simulink model "MK_control_SIL_20200323"  (R2016b)
settings: Solver=ode4  StartTime=0.0  StopTime=inf  FixedStep=0.004  RelTol=1e-7
libraries: simulink x6, simulink_extras x3, etargetslib x1, dspnetwork x1, X_Plane_Communication_Library x1
settings Model: Creator=E6320  LastModifiedBy=user
settings SolverCC: AlgebraicLoopSolver=LineSearch
settings DataIOCC: SaveOutput=off  SignalLogging=off  DSMLogging=off  SaveTime=off

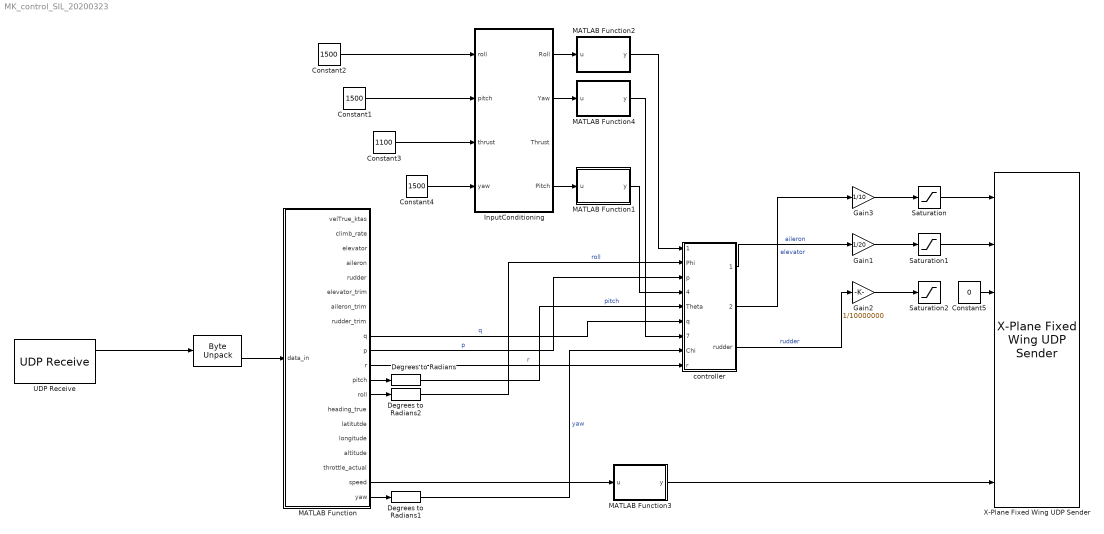
== system MK_control_SIL_20200323 ==
  "     " : etargetslib/Byte Unpack  dimensions={5,[9,21]}  datatypes={'uint8','single'}  byteAlign=1
  Constant1 : Constant  Value=1500
  Constant2 : Constant  Value=1500
  Constant3 : Constant  Value=1100
  Constant4 : Constant  Value=1500
  Constant5 : Constant  Value=0
  Degrees to Radians : simulink_extras/Transformations/Degrees to Radians
  Degrees to Radians1 : simulink_extras/Transformations/Degrees to Radians
  Degrees to Radians2 : simulink_extras/Transformations/Degrees to Radians
  Gain1 : Gain  Gain=1/20
  Gain2 : Gain  Gain=1/10000000
  Gain3 : Gain  Gain=1/10
  InputConditioning : Subsystem
  MATLAB Function : MATLAB Function  TreatAsAtomicUnit=on
  MATLAB Function1 : MATLAB Function  TreatAsAtomicUnit=on
  MATLAB Function2 : MATLAB Function  TreatAsAtomicUnit=on
  MATLAB Function3 : MATLAB Function  TreatAsAtomicUnit=on
  MATLAB Function4 : MATLAB Function  TreatAsAtomicUnit=on
  Saturation : Saturate  UpperLimit=1  LowerLimit=-1
  Saturation1 : Saturate  UpperLimit=1  LowerLimit=-1
  Saturation2 : Saturate  UpperLimit=1  LowerLimit=-1
  UDP Receive : dspnetwork/UDP Receive  localURL='0.0.0.0'  localPort=49005  remoteURL='127.0.0.1'  remotePort=-1  recvBufferSize=8192  dims=761  signalDatatype=uint8  isVarSize=off  showBlockingTime=on  blockingTime=10  sampletime=0.02  blockPlatform=HOST
  X-Plane Fixed Wing UDP Sender : X_Plane_Communication_Library/Fixed Wing/X-Plane Fixed Wing UDP Sender  ip_adress='127.0.0.1'  port_number=49000
  "controller " : Subsystem
  wires:
  UDP Receive/1 -> "     "/1
  "     "/2 -> MATLAB Function/1(data_in)
  Constant3/1 -> InputConditioning/3(thrust)
  Constant4/1 -> InputConditioning/4(yaw)
  Constant2/1 -> InputConditioning/1(roll)
  Constant1/1 -> InputConditioning/2(pitch)
  InputConditioning/4("Pitch ") -> MATLAB Function1/1(u)
  InputConditioning/1(Roll) -> MATLAB Function2/1(u)
  InputConditioning/2(Yaw) -> MATLAB Function4/1(u)
  MATLAB Function/19(speed) -> MATLAB Function3/1(u)
  MATLAB Function3/1(y) -> X-Plane Fixed Wing UDP Sender/7
  MATLAB Function/12(pitch) -> Degrees to Radians/1
  MATLAB Function/13(roll) -> Degrees to Radians2/1
  Saturation/1 -> X-Plane Fixed Wing UDP Sender/1
  Saturation1/1 -> X-Plane Fixed Wing UDP Sender/2
  MATLAB Function2/1(y) -> "controller "/1(PhiCmd)
  MATLAB Function4/1(y) -> "controller "/7(ChiCmd)
  MATLAB Function1/1(y) -> "controller "/4(ThetaCmd)
  MATLAB Function/9(q) -> "controller "/6(q)  "q"
  MATLAB Function/10(p) -> "controller "/3(p)  "p"
  MATLAB Function/11(r) -> "controller "/9(r)  "r"
  Degrees to Radians/1 -> "controller "/5(Theta)  "pitch"
  Degrees to Radians2/1 -> "controller "/2(Phi)  "roll"
  Degrees to Radians1/1 -> "controller "/8(Chi)  "yaw"
  "controller "/1(aileron) -> Gain1/1  "aileron"
  "controller "/3(rudder) -> Gain2/1  "rudder"
  "controller "/2(elevator) -> Gain3/1  "elevator"
  Gain3/1 -> Saturation/1
  Gain1/1 -> Saturation1/1
  Gain2/1 -> Saturation2/1
  MATLAB Function/20(yaw) -> Degrees to Radians1/1
  Constant5/1 -> X-Plane Fixed Wing UDP Sender/3

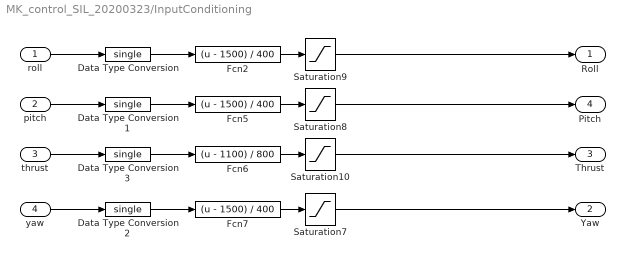
== system MK_control_SIL_20200323/InputConditioning ==
  roll : Inport
  pitch : Inport  Port=2
  thrust : Inport  Port=3
  yaw : Inport  Port=4
  Data Type Conversion{,1..3} (4 alike) : DataTypeConversion  OutDataTypeStr=single
  Fcn2 : Fcn  Expr=(u - 1500) / 400
  Fcn5 : Fcn  Expr=(u - 1500) / 400
  Fcn6 : Fcn  Expr=(u - 1100) / 800
  Fcn7 : Fcn  Expr=(u - 1500) / 400
  Saturation10 : Saturate  UpperLimit=1  LowerLimit=0
  Saturation7 : Saturate  UpperLimit=1  LowerLimit=-1
  Saturation8 : Saturate  UpperLimit=1  LowerLimit=-1
  Saturation9 : Saturate  UpperLimit=1  LowerLimit=-1
  Roll : Outport
  Yaw : Outport  Port=2
  Thrust : Outport  Port=3
  "Pitch " : Outport  Port=4
  wires:
  Saturation10/1 -> Thrust/1
  Saturation9/1 -> Roll/1
  Fcn6/1 -> Saturation10/1
  thrust/1 -> Data Type Conversion3/1
  Fcn2/1 -> Saturation9/1
  Fcn5/1 -> Saturation8/1
  Fcn7/1 -> Saturation7/1
  yaw/1 -> Data Type Conversion2/1
  pitch/1 -> Data Type Conversion1/1
  roll/1 -> Data Type Conversion/1
  Data Type Conversion/1 -> Fcn2/1
  Data Type Conversion1/1 -> Fcn5/1
  Data Type Conversion2/1 -> Fcn7/1
  Data Type Conversion3/1 -> Fcn6/1
  Saturation8/1 -> "Pitch "/1
  Saturation7/1 -> Yaw/1

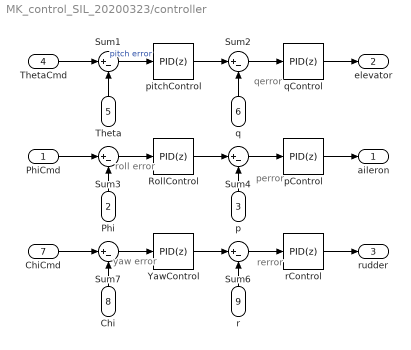
== system MK_control_SIL_20200323/controller  ==
  note: rerror
  note: yaw error
  note: roll error
  note: perror
  note: qerror
  PhiCmd : Inport
  Phi : Inport  Port=2
  p : Inport  Port=3
  ThetaCmd : Inport  Port=4
  Theta : Inport  Port=5
  q : Inport  Port=6
  ChiCmd : Inport  Port=7
  Chi : Inport  Port=8
  r : Inport  Port=9
  RollControl : simulink/Continuous/PID Controller  Controller=PID  TimeDomain=Discrete-time  SampleTime=0.004  IntegratorMethod=Forward Euler  FilterMethod=Forward Euler  Form=Parallel  UseFilter=on  ControllerParametersSource=internal  P=4.82  I=0.5842424242  D=0.401024  N=20.6  InitialConditionSource=internal  InitialConditionForIntegrator=0  InitialConditionForFilter=0  ExternalReset=none  LimitOutput=off  UpperSaturationLimit=inf  LowerSaturationLimit=-inf  LinearizeAsGain=on  AntiWindupMode=none  Kb=1  TrackingMode=off  Kt=1  PParamMin=[]  PParamMax=[]  IParamMin=[]  IParamMax=[]  DParamMin=[]  DParamMax=[]  NParamMin=[]  NParamMax=[]  KbParamMin=[]  KbParamMax=[]  KtParamMin=[]  KtParamMax=[]  POutMin=[]  POutMax=[]  IOutMin=[]  IOutMax=[]  DOutMin=[]  DOutMax=[]  NOutMin=[]  NOutMax=[]  KbOutMin=[]  KbOutMax=[]  KtOutMin=[]  KtOutMax=[]  IntegratorOutMin=[]  IntegratorOutMax=[]  FilterOutMin=[]  FilterOutMax=[]  SumOutMin=[]  SumOutMax=[]  SumI1OutMin=[]  SumI1OutMax=[]  SumI2OutMin=[]  SumI2OutMax=[]  SumI3OutMin=[]  SumI3OutMax=[]  SumDOutMin=[]  SumDOutMax=[]  SaturationOutMin=[]  SaturationOutMax=[]  IntegratorContinuousStateAttributes=''  IntegratorStateMustResolveToSignalObject=off  IntegratorRTWStateStorageClass=Auto  FilterContinuousStateAttributes=''  FilterStateMustResolveToSignalObject=off  FilterRTWStateStorageClass=Auto  DifferentiatorICPrevScaledInput=0  DifferentiatorOutMin=[]  DifferentiatorOutMax=[]
  Sum{1..4,6..7} (6 alike) : Sum  Inputs=|+-
  YawControl : simulink/Continuous/PID Controller  Controller=PID  TimeDomain=Discrete-time  SampleTime=0.004  IntegratorMethod=Forward Euler  FilterMethod=Forward Euler  Form=Parallel  UseFilter=on  ControllerParametersSource=internal  P=17.9  I=36.30831643  D=0.24881  N=3.48  InitialConditionSource=internal  InitialConditionForIntegrator=0  InitialConditionForFilter=0  ExternalReset=none  LimitOutput=off  UpperSaturationLimit=inf  LowerSaturationLimit=-inf  LinearizeAsGain=on  AntiWindupMode=none  Kb=1  TrackingMode=off  Kt=1  PParamMin=[]  PParamMax=[]  IParamMin=[]  IParamMax=[]  DParamMin=[]  DParamMax=[]  NParamMin=[]  NParamMax=[]  KbParamMin=[]  KbParamMax=[]  KtParamMin=[]  KtParamMax=[]  POutMin=[]  POutMax=[]  IOutMin=[]  IOutMax=[]  DOutMin=[]  DOutMax=[]  NOutMin=[]  NOutMax=[]  KbOutMin=[]  KbOutMax=[]  KtOutMin=[]  KtOutMax=[]  IntegratorOutMin=[]  IntegratorOutMax=[]  FilterOutMin=[]  FilterOutMax=[]  SumOutMin=[]  SumOutMax=[]  SumI1OutMin=[]  SumI1OutMax=[]  SumI2OutMin=[]  SumI2OutMax=[]  SumI3OutMin=[]  SumI3OutMax=[]  SumDOutMin=[]  SumDOutMax=[]  SaturationOutMin=[]  SaturationOutMax=[]  IntegratorContinuousStateAttributes=''  IntegratorStateMustResolveToSignalObject=off  IntegratorRTWStateStorageClass=Auto  FilterContinuousStateAttributes=''  FilterStateMustResolveToSignalObject=off  FilterRTWStateStorageClass=Auto  DifferentiatorICPrevScaledInput=0  DifferentiatorOutMin=[]  DifferentiatorOutMax=[]
  pControl : simulink/Continuous/PID Controller  Controller=PID  TimeDomain=Discrete-time  SampleTime=0.004  IntegratorMethod=Forward Euler  FilterMethod=Forward Euler  Form=Parallel  UseFilter=on  ControllerParametersSource=internal  P=0.302  I=2.770642202  D=0.0097546  N=8.07  InitialConditionSource=internal  InitialConditionForIntegrator=0  InitialConditionForFilter=0  ExternalReset=none  LimitOutput=off  UpperSaturationLimit=inf  LowerSaturationLimit=-inf  LinearizeAsGain=on  AntiWindupMode=none  Kb=1  TrackingMode=off  Kt=1  PParamMin=[]  PParamMax=[]  IParamMin=[]  IParamMax=[]  DParamMin=[]  DParamMax=[]  NParamMin=[]  NParamMax=[]  KbParamMin=[]  KbParamMax=[]  KtParamMin=[]  KtParamMax=[]  POutMin=[]  POutMax=[]  IOutMin=[]  IOutMax=[]  DOutMin=[]  DOutMax=[]  NOutMin=[]  NOutMax=[]  KbOutMin=[]  KbOutMax=[]  KtOutMin=[]  KtOutMax=[]  IntegratorOutMin=[]  IntegratorOutMax=[]  FilterOutMin=[]  FilterOutMax=[]  SumOutMin=[]  SumOutMax=[]  SumI1OutMin=[]  SumI1OutMax=[]  SumI2OutMin=[]  SumI2OutMax=[]  SumI3OutMin=[]  SumI3OutMax=[]  SumDOutMin=[]  SumDOutMax=[]  SaturationOutMin=[]  SaturationOutMax=[]  IntegratorContinuousStateAttributes=''  IntegratorStateMustResolveToSignalObject=off  IntegratorRTWStateStorageClass=Auto  FilterContinuousStateAttributes=''  FilterStateMustResolveToSignalObject=off  FilterRTWStateStorageClass=Auto  DifferentiatorICPrevScaledInput=0  DifferentiatorOutMin=[]  DifferentiatorOutMax=[]
  pitchControl : simulink/Continuous/PID Controller  Controller=PID  TimeDomain=Discrete-time  SampleTime=0.004  IntegratorMethod=Forward Euler  FilterMethod=Forward Euler  Form=Parallel  UseFilter=on  ControllerParametersSource=internal  P=5.91  I=5.91  D=0.19503  N=8.24  InitialConditionSource=internal  InitialConditionForIntegrator=0  InitialConditionForFilter=0  ExternalReset=none  LimitOutput=off  UpperSaturationLimit=inf  LowerSaturationLimit=-inf  LinearizeAsGain=on  AntiWindupMode=none  Kb=1  TrackingMode=off  Kt=1  PParamMin=[]  PParamMax=[]  IParamMin=[]  IParamMax=[]  DParamMin=[]  DParamMax=[]  NParamMin=[]  NParamMax=[]  KbParamMin=[]  KbParamMax=[]  KtParamMin=[]  KtParamMax=[]  POutMin=[]  POutMax=[]  IOutMin=[]  IOutMax=[]  DOutMin=[]  DOutMax=[]  NOutMin=[]  NOutMax=[]  KbOutMin=[]  KbOutMax=[]  KtOutMin=[]  KtOutMax=[]  IntegratorOutMin=[]  IntegratorOutMax=[]  FilterOutMin=[]  FilterOutMax=[]  SumOutMin=[]  SumOutMax=[]  SumI1OutMin=[]  SumI1OutMax=[]  SumI2OutMin=[]  SumI2OutMax=[]  SumI3OutMin=[]  SumI3OutMax=[]  SumDOutMin=[]  SumDOutMax=[]  SaturationOutMin=[]  SaturationOutMax=[]  IntegratorContinuousStateAttributes=''  IntegratorStateMustResolveToSignalObject=off  IntegratorRTWStateStorageClass=Auto  FilterContinuousStateAttributes=''  FilterStateMustResolveToSignalObject=off  FilterRTWStateStorageClass=Auto  DifferentiatorICPrevScaledInput=0  DifferentiatorOutMin=[]  DifferentiatorOutMax=[]
  qControl : simulink/Continuous/PID Controller  Controller=PID  TimeDomain=Discrete-time  SampleTime=0.004  IntegratorMethod=Forward Euler  FilterMethod=Forward Euler  Form=Parallel  UseFilter=on  ControllerParametersSource=internal  P=2.96  I=57.14285714  D=0.1702  N=14.4  InitialConditionSource=internal  InitialConditionForIntegrator=0  InitialConditionForFilter=0  ExternalReset=none  LimitOutput=off  UpperSaturationLimit=inf  LowerSaturationLimit=-inf  LinearizeAsGain=on  AntiWindupMode=none  Kb=1  TrackingMode=off  Kt=1  PParamMin=[]  PParamMax=[]  IParamMin=[]  IParamMax=[]  DParamMin=[]  DParamMax=[]  NParamMin=[]  NParamMax=[]  KbParamMin=[]  KbParamMax=[]  KtParamMin=[]  KtParamMax=[]  POutMin=[]  POutMax=[]  IOutMin=[]  IOutMax=[]  DOutMin=[]  DOutMax=[]  NOutMin=[]  NOutMax=[]  KbOutMin=[]  KbOutMax=[]  KtOutMin=[]  KtOutMax=[]  IntegratorOutMin=[]  IntegratorOutMax=[]  FilterOutMin=[]  FilterOutMax=[]  SumOutMin=[]  SumOutMax=[]  SumI1OutMin=[]  SumI1OutMax=[]  SumI2OutMin=[]  SumI2OutMax=[]  SumI3OutMin=[]  SumI3OutMax=[]  SumDOutMin=[]  SumDOutMax=[]  SaturationOutMin=[]  SaturationOutMax=[]  IntegratorContinuousStateAttributes=''  IntegratorStateMustResolveToSignalObject=off  IntegratorRTWStateStorageClass=Auto  FilterContinuousStateAttributes=''  FilterStateMustResolveToSignalObject=off  FilterRTWStateStorageClass=Auto  DifferentiatorICPrevScaledInput=0  DifferentiatorOutMin=[]  DifferentiatorOutMax=[]
  rControl : simulink/Continuous/PID Controller  Controller=PID  TimeDomain=Discrete-time  SampleTime=0.004  IntegratorMethod=Forward Euler  FilterMethod=Forward Euler  Form=Parallel  UseFilter=on  ControllerParametersSource=internal  P=16  I=153.8461538  D=1.5024  N=23.1  InitialConditionSource=internal  InitialConditionForIntegrator=0  InitialConditionForFilter=0  ExternalReset=none  LimitOutput=off  UpperSaturationLimit=inf  LowerSaturationLimit=-inf  LinearizeAsGain=on  AntiWindupMode=none  Kb=1  TrackingMode=off  Kt=1  PParamMin=[]  PParamMax=[]  IParamMin=[]  IParamMax=[]  DParamMin=[]  DParamMax=[]  NParamMin=[]  NParamMax=[]  KbParamMin=[]  KbParamMax=[]  KtParamMin=[]  KtParamMax=[]  POutMin=[]  POutMax=[]  IOutMin=[]  IOutMax=[]  DOutMin=[]  DOutMax=[]  NOutMin=[]  NOutMax=[]  KbOutMin=[]  KbOutMax=[]  KtOutMin=[]  KtOutMax=[]  IntegratorOutMin=[]  IntegratorOutMax=[]  FilterOutMin=[]  FilterOutMax=[]  SumOutMin=[]  SumOutMax=[]  SumI1OutMin=[]  SumI1OutMax=[]  SumI2OutMin=[]  SumI2OutMax=[]  SumI3OutMin=[]  SumI3OutMax=[]  SumDOutMin=[]  SumDOutMax=[]  SaturationOutMin=[]  SaturationOutMax=[]  IntegratorContinuousStateAttributes=''  IntegratorStateMustResolveToSignalObject=off  IntegratorRTWStateStorageClass=Auto  FilterContinuousStateAttributes=''  FilterStateMustResolveToSignalObject=off  FilterRTWStateStorageClass=Auto  DifferentiatorICPrevScaledInput=0  DifferentiatorOutMin=[]  DifferentiatorOutMax=[]
  aileron : Outport
  elevator : Outport  Port=2
  rudder : Outport  Port=3
  wires:
  Sum1/1 -> pitchControl/1  "pitch error"
  ThetaCmd/1 -> Sum1/1
  pitchControl/1 -> Sum2/1
  Sum2/1 -> qControl/1
  qControl/1 -> elevator/1
  Theta/1 -> Sum1/2
  q/1 -> Sum2/2
  Sum3/1 -> RollControl/1
  PhiCmd/1 -> Sum3/1
  RollControl/1 -> Sum4/1
  Sum4/1 -> pControl/1
  Phi/1 -> Sum3/2
  p/1 -> Sum4/2
  Sum7/1 -> YawControl/1
  YawControl/1 -> Sum6/1
  Sum6/1 -> rControl/1
  rControl/1 -> rudder/1
  Chi/1 -> Sum7/2
  r/1 -> Sum6/2
  pControl/1 -> aileron/1
  ChiCmd/1 -> Sum7/1

== matlab function MK_control_SIL_20200323/MATLAB Function1 ==
  data: u input; y output
function y = fcn(u)

y = round(u*100)/100;

== matlab function MK_control_SIL_20200323/MATLAB Function ==
  data: data_in input; velTrue_ktas output; climb_rate output; elevator output; aileron output; rudder output; elevator_trim output; aileron_trim output; rudder_trim output; q output; p output; r output; pitch output; roll output; heading_true output; latitutde output; longitude output; altitude output; throttle_actual output; speed output; yaw output
function [velTrue_ktas, climb_rate,elevator, aileron, rudder, elevator_trim, aileron_trim, rudder_trim, q,p,r, pitch, roll, heading_true, latitutde, longitude, altitude, throttle_actual,speed,yaw]   = fcn(data_in)
% This block supports the Embedded MATLAB subset.
% See the help menu for details. 


velTrue_ktas = data_in(4,1);

climb_rate = data_in(4,2);

elevator = data_in(2,3);
aileron = data_in(3,3);
rudder= data_in(4,3);


elevator_trim= data_in(2,4);
aileron_trim= data_in(3,4);
rudder_trim= data_in(4,4);

q= data_in(2,5);
p= data_in(3,5);
r= data_in(4,5);
yaw = data_in(6,3);

pitch= data_in(2,6);
roll= data_in(3,6);
heading_true= data_in(4,6);

latitutde= data_in(2,7);
longitude= data_in(3,7);

altitude= data_in(4,7);
throttle_actual = data_in(2,8);
speed = data_in(2,2);

== matlab function MK_control_SIL_20200323/MATLAB Function2 ==
  data: u input; y output
function y = fcn(u)

y = round(u*100)/100;

== matlab function MK_control_SIL_20200323/MATLAB Function3 ==
  data: u input; y output
function y = fcn(u)
if(u<=0.044)
y = 0.7;
else
    y=0.2
end

== matlab function MK_control_SIL_20200323/MATLAB Function4 ==
  data: u input; y output
function y = fcn(u)

y = round(u*100)/100;
